simulink model "sl_robot_sincrono_control_postura"  (R2016b)
settings: Solver=VariableStepAuto  StartTime=0.0  StopTime=tsim  RelTol=1e-3
values from neighbouring files (symbols this model uses):
  ang_ref = in(3)    [control_postura.m]    (also in pruebas_control_P2.m = 3.14159265359)
  d = (a*x + b*y + c*1)/(sqrt(a^2 + b^2))    [control_linea.m]    (also in pruebas_control_P2.m = 0)
  omega_sat = [-0.2618 0.2618]    [pruebas_control_P2.m]
  pos_init = [0;0;0]    [pruebas_control_P2.m]
  px_ref = in(1)    [control_postura.m]    (also in pruebas_control_P2.m = 15)
  py_ref = in(2)    [control_postura.m]    (also in pruebas_control_P2.m = 5)
  tetha_d_sat = [-0.75 0.75]    [pruebas_control_P2.m]
  Tm = 0.01    [control_tray.m]    (also in pruebas_control_P2.m)
settings Model: Creator=marrcogrova  LastModifiedBy=marrcogrova

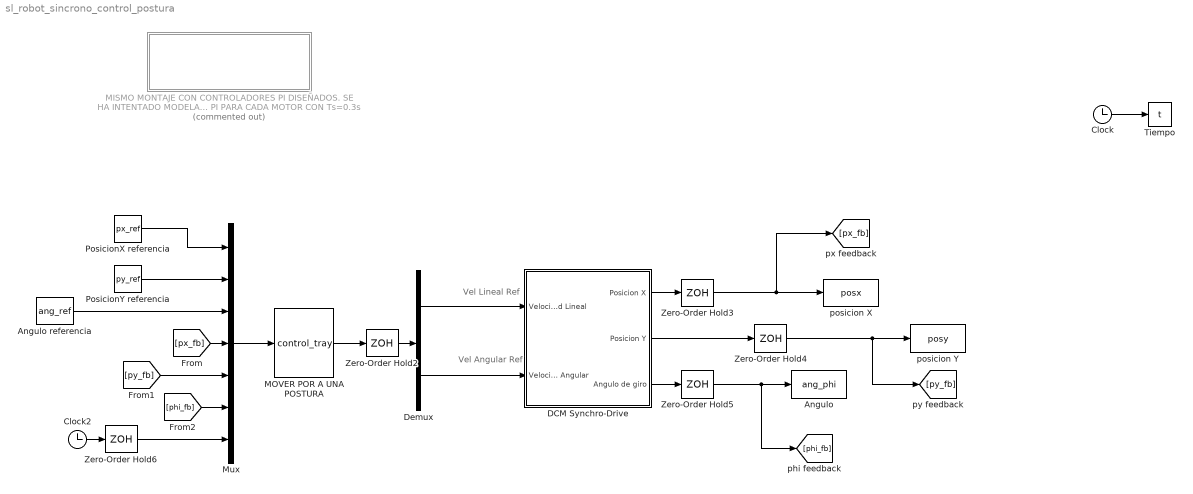
== system sl_robot_sincrono_control_postura ==
  note: Vel Lineal Ref
  note: Vel Angular Ref
  Angulo : ToWorkspace  VariableName=ang_phi  SampleTime=-1
  "Angulo referencia " : Constant  Value=ang_ref
  Clock : Clock
  Clock2 : Clock
  DCM Synchro-Drive : Subsystem
  Demux : Demux  Outputs=2
  MISMO MONTAJE CON CONTROLADORES PI DISEÑADOS. SE HA INTENTADO MODELAR LOS MOTORES Y DISEÑAR UN PI PARA CADA MOTOR CON Ts=0.3s : Subsystem  Commented=on
  MOVER POR A UNA POSTURA : MATLABFcn  MATLABFcn=control_tray  OutputDimensions=2
  Mux : Mux  Inputs=7
  PosicionX referencia : Constant  Value=px_ref
  PosicionY referencia : Constant  Value=py_ref
  Tiempo : ToWorkspace  VariableName=t  SampleTime=-1
  Zero-Order Hold{2..6} (5 alike) : ZeroOrderHold  SampleTime=Tm
  posicion X : ToWorkspace  VariableName=posx  SampleTime=-1
  posicion Y : ToWorkspace  VariableName=posy  SampleTime=-1
  wires:
  Clock/1 -> Tiempo/1
  DCM Synchro-Drive/2(Posicion Y) -> Zero-Order Hold4/1
  MOVER POR A UNA POSTURA/1 -> Zero-Order Hold2/1
  Mux/1 -> MOVER POR A UNA POSTURA/1
  DCM Synchro-Drive/3(Angulo de giro) -> Zero-Order Hold5/1
  [phi_fb] -> Mux/6
  [py_fb] -> Mux/5
  [px_fb] -> Mux/4
  Demux/1 -> DCM Synchro-Drive/1(Velocidad Lineal)
  Demux/2 -> DCM Synchro-Drive/2(Velocidad Angular)
  Zero-Order Hold2/1 -> Demux/1
  Zero-Order Hold3/1 -> [px_fb], posicion X/1
  DCM Synchro-Drive/1(Posicion X) -> Zero-Order Hold3/1
  Zero-Order Hold4/1 -> posicion Y/1, [py_fb]
  Zero-Order Hold5/1 -> [phi_fb], Angulo/1
  Clock2/1 -> Zero-Order Hold6/1
  Zero-Order Hold6/1 -> Mux/7
  PosicionX referencia/1 -> Mux/1
  PosicionY referencia/1 -> Mux/2
  "Angulo referencia "/1 -> Mux/3

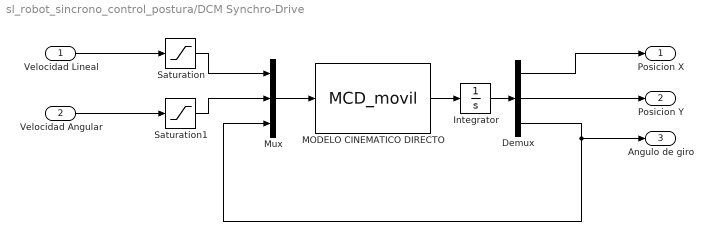
== system sl_robot_sincrono_control_postura/DCM Synchro-Drive ==
  Velocidad Lineal : Inport
  Velocidad Angular : Inport  Port=2
  Demux : Demux  Outputs=3
  Integrator : Integrator  InitialCondition=pos_init
  MODELO CINEMATICO DIRECTO : MATLABFcn  MATLABFcn=MCD_movil  OutputDimensions=3
  Mux : Mux  Inputs=3
  Saturation : Saturate  UpperLimit=tetha_d_sat(2)  LowerLimit=tetha_d_sat(1)
  Saturation1 : Saturate  UpperLimit=omega_sat(2)  LowerLimit=omega_sat(1)
  Posicion X : Outport
  Posicion Y : Outport  Port=2
  Angulo de giro : Outport  Port=3
  wires:
  Integrator/1 -> Demux/1
  Demux/3 -> Angulo de giro/1, Mux/3
  Demux/1 -> Posicion X/1
  Demux/2 -> Posicion Y/1
  Mux/1 -> MODELO CINEMATICO DIRECTO/1
  MODELO CINEMATICO DIRECTO/1 -> Integrator/1
  Velocidad Lineal/1 -> Saturation/1
  Saturation/1 -> Mux/1
  Saturation1/1 -> Mux/2
  Velocidad Angular/1 -> Saturation1/1

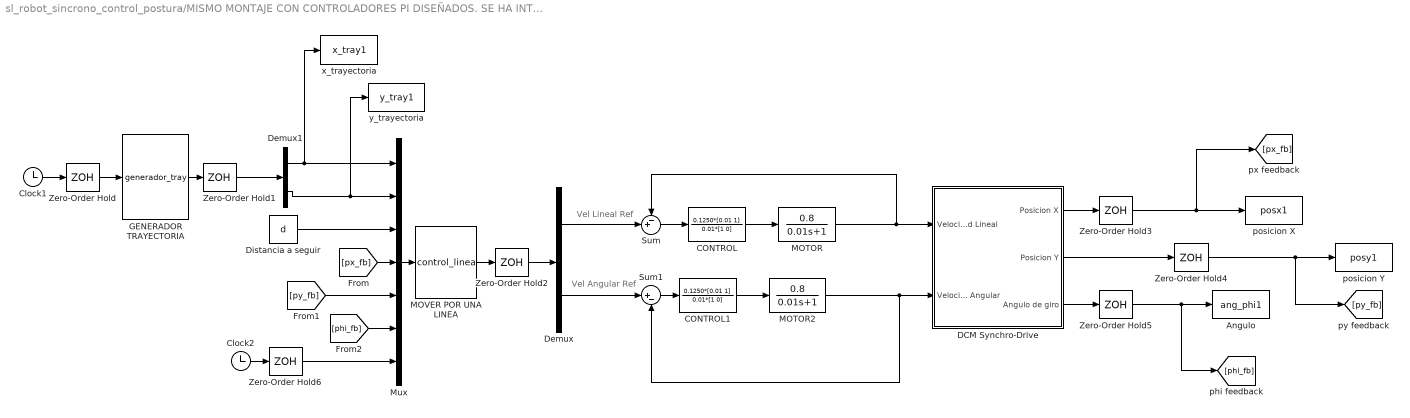
== system sl_robot_sincrono_control_postura/MISMO MONTAJE CON CONTROLADORES PI DISEÑADOS. SE HA INTENTADO MODELAR LOS MOTORES Y DISEÑAR UN PI PARA CADA MOTOR CON Ts=0.3s ==
  note: Vel Lineal Ref
  note: Vel Angular Ref
  Angulo : ToWorkspace  VariableName=ang_phi1  SampleTime=-1
  CONTROL : TransferFcn  Numerator=0.1250*[0.01 1]  Denominator=0.01*[1 0]
  CONTROL1 : TransferFcn  Numerator=0.1250*[0.01 1]  Denominator=0.01*[1 0]
  Clock1 : Clock
  Clock2 : Clock
  DCM Synchro-Drive : Subsystem
  Demux : Demux  Outputs=2
  Demux1 : Demux  Outputs=2
  Distancia a seguir : Constant  Value=d
  GENERADOR TRAYECTORIA : MATLABFcn  MATLABFcn=generador_tray  OutputDimensions=2
  MOTOR : TransferFcn  Numerator=0.8  Denominator=[0.01 1]
  MOTOR2 : TransferFcn  Numerator=0.8  Denominator=[0.01 1]
  MOVER POR UNA LINEA : MATLABFcn  MATLABFcn=control_linea  OutputDimensions=2
  Mux : Mux  Inputs=7
  Sum : Sum  Inputs=-+|
  Sum1 : Sum  Inputs=|+-
  Zero-Order Hold{,1..6} (7 alike) : ZeroOrderHold  SampleTime=Tm
  posicion X : ToWorkspace  VariableName=posx1  SampleTime=-1
  posicion Y : ToWorkspace  VariableName=posy1  SampleTime=-1
  x_trayectoria : ToWorkspace  VariableName=x_tray1  SampleTime=Tm
  y_trayectoria : ToWorkspace  VariableName=y_tray1  SampleTime=Tm
  wires:
  MOVER POR UNA LINEA/1 -> Zero-Order Hold2/1
  Demux/1 -> Sum/2
  Sum/1 -> CONTROL/1
  Demux/2 -> Sum1/1
  Sum1/1 -> CONTROL1/1
  MOTOR2/1 -> DCM Synchro-Drive/2(Velocidad Angular), Sum1/2
  MOTOR/1 -> DCM Synchro-Drive/1(Velocidad Lineal), Sum/1
  CONTROL/1 -> MOTOR/1
  CONTROL1/1 -> MOTOR2/1
  Demux1/1 -> Mux/1, x_trayectoria/1
  Demux1/2 -> y_trayectoria/1, Mux/2
  [phi_fb] -> Mux/6
  [py_fb] -> Mux/5
  [px_fb] -> Mux/4
  Distancia a seguir/1 -> Mux/3
  Zero-Order Hold/1 -> GENERADOR TRAYECTORIA/1
  GENERADOR TRAYECTORIA/1 -> Zero-Order Hold1/1
  Zero-Order Hold1/1 -> Demux1/1
  Clock2/1 -> Zero-Order Hold6/1
  Zero-Order Hold6/1 -> Mux/7
  Mux/1 -> MOVER POR UNA LINEA/1
  DCM Synchro-Drive/2(Posicion Y) -> Zero-Order Hold4/1
  Zero-Order Hold3/1 -> [px_fb], posicion X/1
  Zero-Order Hold4/1 -> posicion Y/1, [py_fb]
  Zero-Order Hold5/1 -> [phi_fb], Angulo/1
  DCM Synchro-Drive/3(Angulo de giro) -> Zero-Order Hold5/1
  DCM Synchro-Drive/1(Posicion X) -> Zero-Order Hold3/1
  Zero-Order Hold2/1 -> Demux/1
  Clock1/1 -> Zero-Order Hold/1

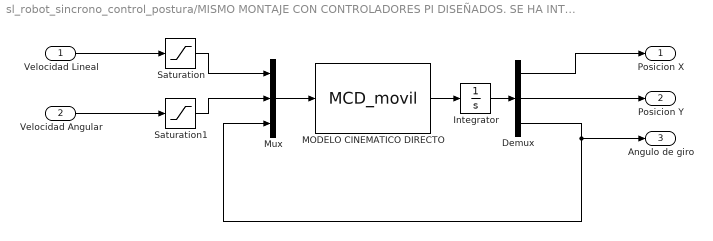
== system sl_robot_sincrono_control_postura/MISMO MONTAJE CON CONTROLADORES PI DISEÑADOS. SE HA INTENTADO MODELAR LOS MOTORES Y DISEÑAR UN PI PARA CADA MOTOR CON Ts=0.3s/DCM Synchro-Drive ==
  Velocidad Lineal : Inport
  Velocidad Angular : Inport  Port=2
  Demux : Demux  Outputs=3
  Integrator : Integrator  InitialCondition=pos_init
  MODELO CINEMATICO DIRECTO : MATLABFcn  MATLABFcn=MCD_movil  OutputDimensions=3
  Mux : Mux  Inputs=3
  Saturation : Saturate  UpperLimit=tetha_d_sat(2)  LowerLimit=tetha_d_sat(1)
  Saturation1 : Saturate  UpperLimit=omega_sat(2)  LowerLimit=omega_sat(1)
  Posicion X : Outport
  Posicion Y : Outport  Port=2
  Angulo de giro : Outport  Port=3
  wires:
  Integrator/1 -> Demux/1
  Demux/3 -> Angulo de giro/1, Mux/3
  Demux/1 -> Posicion X/1
  Demux/2 -> Posicion Y/1
  Mux/1 -> MODELO CINEMATICO DIRECTO/1
  MODELO CINEMATICO DIRECTO/1 -> Integrator/1
  Velocidad Lineal/1 -> Saturation/1
  Saturation/1 -> Mux/1
  Saturation1/1 -> Mux/2
  Velocidad Angular/1 -> Saturation1/1
